simulink model "testforward"  (R2015a)
settings: Solver=ode3  StartTime=0.0  StopTime=10.0  RelTol=1e-3
undefined symbols (not defined in the file): X, Y
libraries: robotlib x3
settings Model: Creator=Kelan  LastModifiedBy=Kelan
settings OptimizationCC: EnhancedBackFolding=on

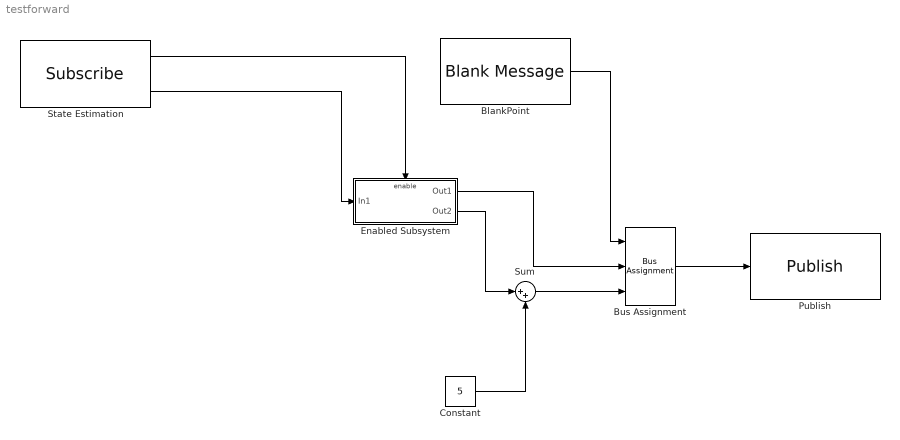
== system testforward ==
  BlankPoint : robotlib/Blank Message  SourceLibraryInfo=This block requires Robotics System Toolbox  messageType=geometry_msgs/Point  SampleTime=inf
  Bus Assignment : BusAssignment  AssignedSignals=X,Y
  Constant : Constant  Value=5
  Enabled Subsystem : Subsystem  TreatAsAtomicUnit=on
  Publish : robotlib/Publish  SourceLibraryInfo=This block requires Robotics System Toolbox  topicSource=Specify your own  topic=/Goal  messageType=geometry_msgs/Point  messageQueueLength=1
  State Estimation : robotlib/Subscribe  SourceLibraryInfo=This block requires Robotics System Toolbox  topicSource=Specify your own  topic=/state  messageType=geometry_msgs/Point  sampleTime=-1  messageQueueLength=1
  Sum : Sum  Inputs=|++
  wires:
  State Estimation/1 -> Enabled Subsystem/Enable
  State Estimation/2 -> Enabled Subsystem/1(In1)
  BlankPoint/1 -> Bus Assignment/1
  Bus Assignment/1 -> Publish/1
  Enabled Subsystem/1(Out1) -> Bus Assignment/2
  Sum/1 -> Bus Assignment/3
  Constant/1 -> Sum/2
  Enabled Subsystem/2(Out2) -> Sum/1

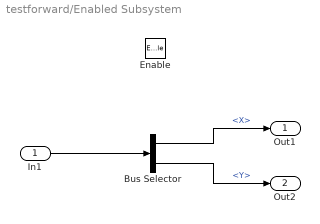
== system testforward/Enabled Subsystem ==
  In1 : Inport
  Enable : EnablePort
  Bus Selector : BusSelector  OutputSignals=X,Y
  Out1 : Outport
  Out2 : Outport  Port=2
  wires:
  In1/1 -> Bus Selector/1
  Bus Selector/1 -> Out1/1  "<X>"
  Bus Selector/2 -> Out2/1  "<Y>"
